simulink model "Simulink_Propusleur_P1"  (R2019b)
settings: Solver=ode1  StartTime=0.0  StopTime=0.1  FixedStep=1e-4  RelTol=1e-3
values from neighbouring files (symbols this model uses):
  f = 6.52e-6    (= 6.52e-06)    [Script_Propulseur_P1.m]
  J = (Kem*Kem*tauEm)/Rm    (= 1.1664e-07)    [Script_Propulseur_P1.m]
  Kem = 2.7e-3    (= 0.0027)    [Script_Propulseur_P1.m]
  Lm = 2e-3    (= 0.002)    [Script_Propulseur_P1.m]
  Rm = 1    [Script_Propulseur_P1.m]
settings Model: Creator=titil  LastModifiedBy=titil

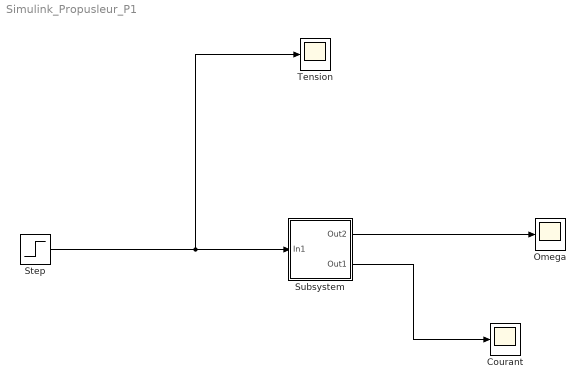
== system Simulink_Propusleur_P1 ==
  Courant : Scope
  Omega : Scope
  Step : Step  Time=0  After=7.2  SampleTime=0
  Subsystem : Subsystem
  Tension : Scope
  wires:
  Step/1 -> Subsystem/1(In1), Tension/1
  Subsystem/2(Out1) -> Courant/1
  Subsystem/1(Out2) -> Omega/1

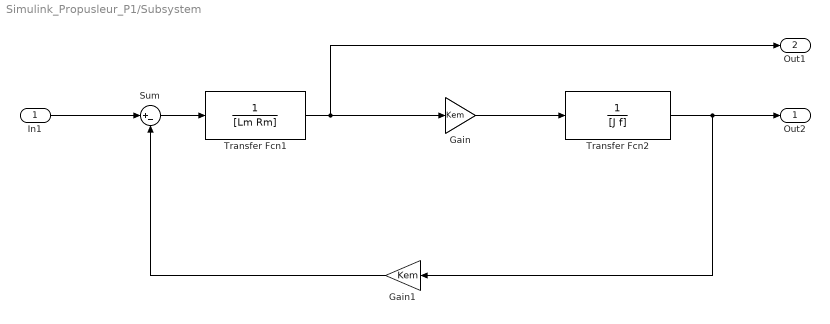
== system Simulink_Propusleur_P1/Subsystem ==
  In1 : Inport
  Gain : Gain  Gain=Kem
  Gain1 : Gain  Gain=Kem
  Sum : Sum  Inputs=|+-
  Transfer Fcn1 : TransferFcn  Denominator=[Lm Rm]
  Transfer Fcn2 : TransferFcn  Denominator=[J f]
  Out2 : Outport
  Out1 : Outport  Port=2
  wires:
  Sum/1 -> Transfer Fcn1/1
  Gain1/1 -> Sum/2
  Transfer Fcn2/1 -> Out2/1, Gain1/1
  Transfer Fcn1/1 -> Out1/1, Gain/1
  Gain/1 -> Transfer Fcn2/1
  In1/1 -> Sum/1
